simulink model "v08_fourbit_add"  (R2019b)
settings: Solver=FixedStepAuto  StartTime=0.0  StopTime=inf  FixedStep=1  MaxStep=1  RelTol=1e-3
libraries: simulink x8
settings Model: Creator=MARAT  LastModifiedBy=Marat
settings SFSimCC: CustomCodeUndefinedFunction=UseInterfaceOnly

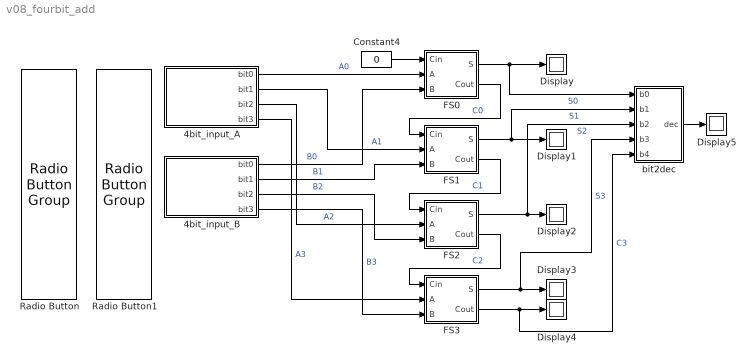
== system v08_fourbit_add ==
  4bit_input_A : Subsystem
      mask Display: image('images\sansA.png'); % Use "Edit Image" on toolstrip to change.
  4bit_input_B : Subsystem
      mask Display: image('images\sansB.png'); % Use "Edit Image" on toolstrip to change.
  Constant4 : Constant  Value=0  OutDataTypeStr=boolean
  Display{,1..5} (6 alike) : Display
  FS0 : Subsystem
  FS1 : Subsystem
  FS2 : Subsystem
  FS3 : Subsystem
  Radio Button : RadioButtonGroup  SelectedLabel=0
      settings: Values={{'0', '1', '2', '3', '4', '5', '6', '7', '8', '9', '10', '11', '12', '13', '14', '15'}, [0 1 2 3 4 5 6 7 8 9 10 11 12 13 14 15]}
  Radio Button1 : RadioButtonGroup  SelectedLabel=0
      settings: Values={{'0', '1', '2', '3', '4', '5', '6', '7', '8', '9', '10', '11', '12', '13', '14', '15'}, [0 1 2 3 4 5 6 7 8 9 10 11 12 13 14 15]}
  bit2dec : Subsystem
  wires:
  Constant4/1 -> FS0/1(Cin)
  FS0/1(S) -> bit2dec/1(b0), Display/1  "S0"
  FS0/2(Cout) -> FS1/1(Cin)  "С0"
  FS1/2(Cout) -> FS2/1(Cin)  "С1"
  FS2/2(Cout) -> FS3/1(Cin)  "С2"
  FS1/1(S) -> bit2dec/2(b1), Display1/1  "S1"
  FS2/1(S) -> bit2dec/3(b2), Display2/1  "S2"
  FS3/1(S) -> bit2dec/4(b3), Display3/1  "S3"
  FS3/2(Cout) -> Display4/1, bit2dec/5(b4)  "С3"
  4bit_input_A/1(bit0) -> FS0/2(A)  "A0"
  4bit_input_A/2(bit1) -> FS1/2(A)  "A1"
  4bit_input_A/3(bit2) -> FS2/2(A)  "A2"
  4bit_input_A/4(bit3) -> FS3/2(A)  "A3"
  4bit_input_B/1(bit0) -> FS0/3(B)  "B0"
  4bit_input_B/2(bit1) -> FS1/3(B)  "B1"
  4bit_input_B/3(bit2) -> FS2/3(B)  "B2"
  4bit_input_B/4(bit3) -> FS3/3(B)  "B3"
  bit2dec/1(dec) -> Display5/1

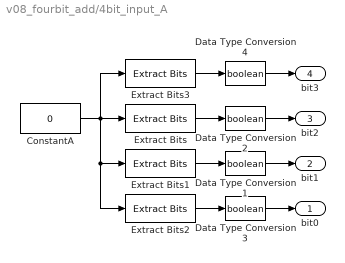
== system v08_fourbit_add/4bit_input_A ==
  ConstantA : Constant  Value=0  OutMin=0  OutMax=15  OutDataTypeStr=uint8
  Data Type Conversion{1..4} (4 alike) : DataTypeConversion  OutDataTypeStr=boolean
  Extract Bits : simulink/Logic and Bit Operations/Extract Bits  bitsToExtract=Range of bits  numBits=8  bitIdxRange=2  outScalingMode=Treat bit field as an integer
      settings: SourceProductName=Simulink
  Extract Bits1 : simulink/Logic and Bit Operations/Extract Bits  bitsToExtract=Range of bits  numBits=8  bitIdxRange=1  outScalingMode=Treat bit field as an integer
      settings: SourceProductName=Simulink
  Extract Bits2 : simulink/Logic and Bit Operations/Extract Bits  bitsToExtract=Range of bits  numBits=8  bitIdxRange=0  outScalingMode=Treat bit field as an integer
      settings: SourceProductName=Simulink
  Extract Bits3 : simulink/Logic and Bit Operations/Extract Bits  bitsToExtract=Range of bits  numBits=8  bitIdxRange=3  outScalingMode=Treat bit field as an integer
      settings: SourceProductName=Simulink
  bit0 : Outport
  bit1 : Outport  Port=2
  bit2 : Outport  Port=3
  bit3 : Outport  Port=4
  wires:
  ConstantA/1 -> Extract Bits3/1, Extract Bits2/1, Extract Bits1/1, Extract Bits/1
  Extract Bits/1 -> Data Type Conversion2/1
  Extract Bits1/1 -> Data Type Conversion1/1
  Extract Bits2/1 -> Data Type Conversion3/1
  Data Type Conversion2/1 -> bit2/1
  Data Type Conversion1/1 -> bit1/1
  Data Type Conversion3/1 -> bit0/1
  Data Type Conversion4/1 -> bit3/1
  Extract Bits3/1 -> Data Type Conversion4/1

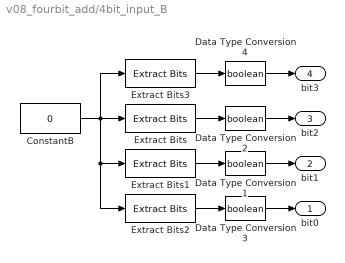
== system v08_fourbit_add/4bit_input_B ==
  ConstantB : Constant  Value=0  OutMin=0  OutMax=15  OutDataTypeStr=uint8
  Data Type Conversion{1..4} (4 alike) : DataTypeConversion  OutDataTypeStr=boolean
  Extract Bits : simulink/Logic and Bit Operations/Extract Bits  bitsToExtract=Range of bits  numBits=8  bitIdxRange=2  outScalingMode=Treat bit field as an integer
      settings: SourceProductName=Simulink
  Extract Bits1 : simulink/Logic and Bit Operations/Extract Bits  bitsToExtract=Range of bits  numBits=8  bitIdxRange=1  outScalingMode=Treat bit field as an integer
      settings: SourceProductName=Simulink
  Extract Bits2 : simulink/Logic and Bit Operations/Extract Bits  bitsToExtract=Range of bits  numBits=8  bitIdxRange=0  outScalingMode=Treat bit field as an integer
      settings: SourceProductName=Simulink
  Extract Bits3 : simulink/Logic and Bit Operations/Extract Bits  bitsToExtract=Range of bits  numBits=8  bitIdxRange=3  outScalingMode=Treat bit field as an integer
      settings: SourceProductName=Simulink
  bit0 : Outport
  bit1 : Outport  Port=2
  bit2 : Outport  Port=3
  bit3 : Outport  Port=4
  wires:
  Extract Bits3/1 -> Data Type Conversion4/1
  Data Type Conversion4/1 -> bit3/1
  Data Type Conversion3/1 -> bit0/1
  Data Type Conversion1/1 -> bit1/1
  Data Type Conversion2/1 -> bit2/1
  Extract Bits2/1 -> Data Type Conversion3/1
  Extract Bits1/1 -> Data Type Conversion1/1
  Extract Bits/1 -> Data Type Conversion2/1
  ConstantB/1 -> Extract Bits/1, Extract Bits1/1, Extract Bits2/1, Extract Bits3/1

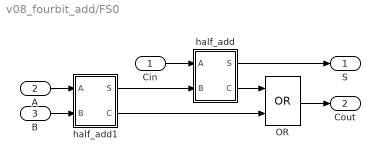
== system v08_fourbit_add/FS0 ==
  Cin : Inport
  A : Inport  Port=2
  B : Inport  Port=3
  OR : Logic  Operator=OR  AllPortsSameDT=off  OutDataTypeStr=boolean
  half_add : Subsystem
  half_add1 : Subsystem
  S : Outport
  Cout : Outport  Port=2
  wires:
  half_add/1(S) -> S/1
  A/1 -> half_add1/1(A)
  half_add/2(C) -> OR/1
  half_add1/1(S) -> half_add/2(B)
  B/1 -> half_add1/2(B)
  Cin/1 -> half_add/1(A)
  OR/1 -> Cout/1
  half_add1/2(C) -> OR/2

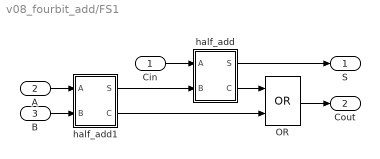
== system v08_fourbit_add/FS1 ==
  Cin : Inport
  A : Inport  Port=2
  B : Inport  Port=3
  OR : Logic  Operator=OR  AllPortsSameDT=off  OutDataTypeStr=boolean
  half_add : Subsystem
  half_add1 : Subsystem
  S : Outport
  Cout : Outport  Port=2
  wires:
  half_add1/2(C) -> OR/2
  OR/1 -> Cout/1
  Cin/1 -> half_add/1(A)
  B/1 -> half_add1/2(B)
  half_add1/1(S) -> half_add/2(B)
  half_add/2(C) -> OR/1
  A/1 -> half_add1/1(A)
  half_add/1(S) -> S/1

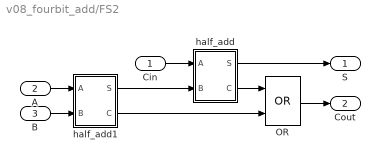
== system v08_fourbit_add/FS2 ==
  Cin : Inport
  A : Inport  Port=2
  B : Inport  Port=3
  OR : Logic  Operator=OR  AllPortsSameDT=off  OutDataTypeStr=boolean
  half_add : Subsystem
  half_add1 : Subsystem
  S : Outport
  Cout : Outport  Port=2
  wires:
  half_add/1(S) -> S/1
  A/1 -> half_add1/1(A)
  half_add/2(C) -> OR/1
  half_add1/1(S) -> half_add/2(B)
  B/1 -> half_add1/2(B)
  Cin/1 -> half_add/1(A)
  OR/1 -> Cout/1
  half_add1/2(C) -> OR/2

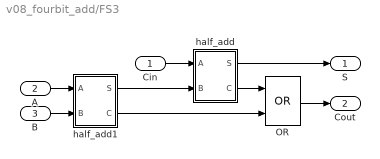
== system v08_fourbit_add/FS3 ==
  Cin : Inport
  A : Inport  Port=2
  B : Inport  Port=3
  OR : Logic  Operator=OR  AllPortsSameDT=off  OutDataTypeStr=boolean
  half_add : Subsystem
  half_add1 : Subsystem
  S : Outport
  Cout : Outport  Port=2
  wires:
  half_add1/2(C) -> OR/2
  OR/1 -> Cout/1
  Cin/1 -> half_add/1(A)
  B/1 -> half_add1/2(B)
  half_add1/1(S) -> half_add/2(B)
  half_add/2(C) -> OR/1
  A/1 -> half_add1/1(A)
  half_add/1(S) -> S/1

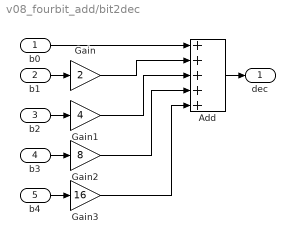
== system v08_fourbit_add/bit2dec ==
  b0 : Inport
  b1 : Inport  Port=2
  b2 : Inport  Port=3
  b3 : Inport  Port=4
  b4 : Inport  Port=5
  Add : Sum  Inputs=+++++
  Gain : Gain  Gain=2
  Gain1 : Gain  Gain=4
  Gain2 : Gain  Gain=8
  Gain3 : Gain  Gain=16
  dec : Outport
  wires:
  b1/1 -> Gain/1
  b3/1 -> Gain2/1
  b2/1 -> Gain1/1
  b0/1 -> Add/1
  Add/1 -> dec/1
  Gain/1 -> Add/2
  Gain1/1 -> Add/3
  Gain2/1 -> Add/4
  b4/1 -> Gain3/1
  Gain3/1 -> Add/5

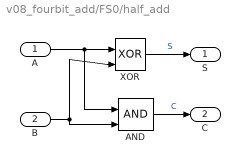
== system v08_fourbit_add/FS0/half_add ==
  A : Inport
  B : Inport  Port=2
  AND : Logic  IconShape=distinctive  AllPortsSameDT=off  OutDataTypeStr=boolean
  XOR : Logic  Operator=XOR  IconShape=distinctive  AllPortsSameDT=off  OutDataTypeStr=boolean
  S : Outport
  C : Outport  Port=2
  wires:
  XOR/1 -> S/1  "S"
  B/1 -> AND/2, XOR/2
  A/1 -> AND/1, XOR/1
  AND/1 -> C/1  "C"

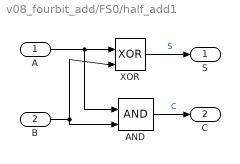
== system v08_fourbit_add/FS0/half_add1 ==
  A : Inport
  B : Inport  Port=2
  AND : Logic  IconShape=distinctive  AllPortsSameDT=off  OutDataTypeStr=boolean
  XOR : Logic  Operator=XOR  IconShape=distinctive  AllPortsSameDT=off  OutDataTypeStr=boolean
  S : Outport
  C : Outport  Port=2
  wires:
  AND/1 -> C/1  "C"
  A/1 -> XOR/1, AND/1
  B/1 -> XOR/2, AND/2
  XOR/1 -> S/1  "S"

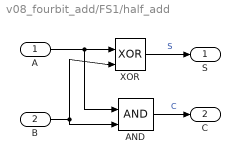
== system v08_fourbit_add/FS1/half_add ==
  A : Inport
  B : Inport  Port=2
  AND : Logic  IconShape=distinctive  AllPortsSameDT=off  OutDataTypeStr=boolean
  XOR : Logic  Operator=XOR  IconShape=distinctive  AllPortsSameDT=off  OutDataTypeStr=boolean
  S : Outport
  C : Outport  Port=2
  wires:
  AND/1 -> C/1  "C"
  A/1 -> XOR/1, AND/1
  B/1 -> XOR/2, AND/2
  XOR/1 -> S/1  "S"

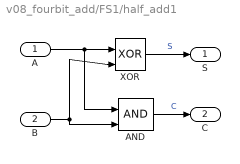
== system v08_fourbit_add/FS1/half_add1 ==
  A : Inport
  B : Inport  Port=2
  AND : Logic  IconShape=distinctive  AllPortsSameDT=off  OutDataTypeStr=boolean
  XOR : Logic  Operator=XOR  IconShape=distinctive  AllPortsSameDT=off  OutDataTypeStr=boolean
  S : Outport
  C : Outport  Port=2
  wires:
  XOR/1 -> S/1  "S"
  B/1 -> AND/2, XOR/2
  A/1 -> AND/1, XOR/1
  AND/1 -> C/1  "C"

== system v08_fourbit_add/FS2/half_add ==
  A : Inport
  B : Inport  Port=2
  AND : Logic  IconShape=distinctive  AllPortsSameDT=off  OutDataTypeStr=boolean
  XOR : Logic  Operator=XOR  IconShape=distinctive  AllPortsSameDT=off  OutDataTypeStr=boolean
  S : Outport
  C : Outport  Port=2
  wires:
  XOR/1 -> S/1  "S"
  B/1 -> AND/2, XOR/2
  A/1 -> AND/1, XOR/1
  AND/1 -> C/1  "C"

== system v08_fourbit_add/FS2/half_add1 ==
  A : Inport
  B : Inport  Port=2
  AND : Logic  IconShape=distinctive  AllPortsSameDT=off  OutDataTypeStr=boolean
  XOR : Logic  Operator=XOR  IconShape=distinctive  AllPortsSameDT=off  OutDataTypeStr=boolean
  S : Outport
  C : Outport  Port=2
  wires:
  AND/1 -> C/1  "C"
  A/1 -> XOR/1, AND/1
  B/1 -> XOR/2, AND/2
  XOR/1 -> S/1  "S"

== system v08_fourbit_add/FS3/half_add ==
  A : Inport
  B : Inport  Port=2
  AND : Logic  IconShape=distinctive  AllPortsSameDT=off  OutDataTypeStr=boolean
  XOR : Logic  Operator=XOR  IconShape=distinctive  AllPortsSameDT=off  OutDataTypeStr=boolean
  S : Outport
  C : Outport  Port=2
  wires:
  AND/1 -> C/1  "C"
  A/1 -> XOR/1, AND/1
  B/1 -> XOR/2, AND/2
  XOR/1 -> S/1  "S"

== system v08_fourbit_add/FS3/half_add1 ==
  A : Inport
  B : Inport  Port=2
  AND : Logic  IconShape=distinctive  AllPortsSameDT=off  OutDataTypeStr=boolean
  XOR : Logic  Operator=XOR  IconShape=distinctive  AllPortsSameDT=off  OutDataTypeStr=boolean
  S : Outport
  C : Outport  Port=2
  wires:
  XOR/1 -> S/1  "S"
  B/1 -> AND/2, XOR/2
  A/1 -> AND/1, XOR/1
  AND/1 -> C/1  "C"
